simulink model "StateSpaceControl"  (R2023b)
settings: Solver=VariableStepAuto  StartTime=0.0  StopTime=20  RelTol=1e-3
values from neighbouring files (symbols this model uses):
  Time = 0:Delta:20    [Animation.m]    (also in Animation2.m; Animation3.m)
undefined symbols (not defined in the file or in its folder): A, B, C, Continuous, D, K_LQR
libraries: ctrlSharedLib x1
settings Model: Creator=BenWo  LastModifiedBy=BenWo

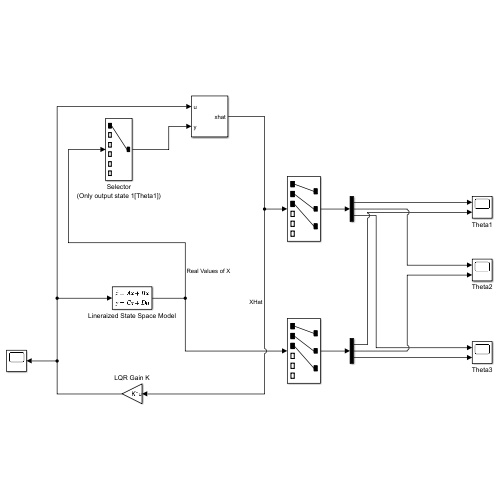
[thumbnail: Simulink's stored preview of the top-level diagram]
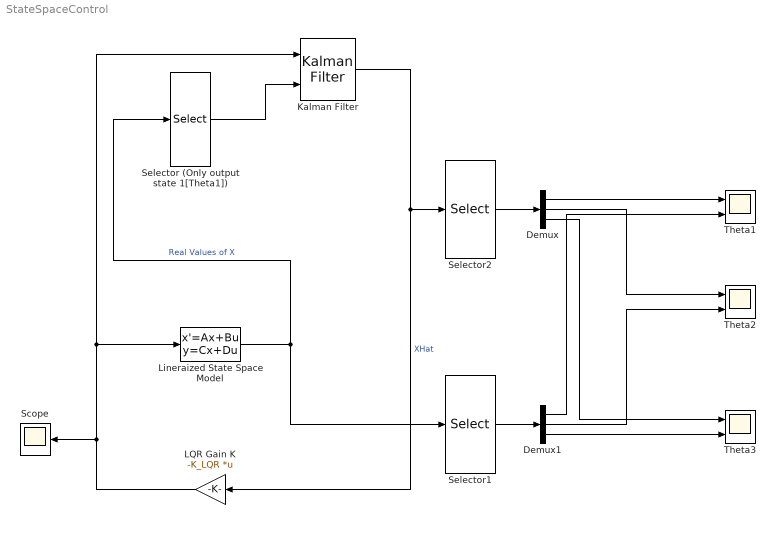
== system StateSpaceControl ==
  Demux : Demux  Outputs=3
  Demux1 : Demux  Outputs=3
  Kalman Filter : ctrlSharedLib/Kalman Filter  TimeDomain=Continuous-Time  UseCurrentEstimator=on  ModelSource=Individual A, B, C, D matrices  ModelSourceVariable=ss(0.95,1,1,0,1)  A=A  B=B  C=C  D=D  NumberOfStates=1  NumberOfInputs=1  NumberOfOutputs=1  InitialEstimateSource=Dialog  X0=0  P0=10  UseK=off  UseGH=off  NumberOfProcessNoiseInputs=1  G=1  TimeInvariantG=on  H=0  TimeInvariantH=on  Q=LQ  TimeInvariantQ=on  R=1  TimeInvariantR=on  N=0  TimeInvariantN=on  AddInputPort=on  AddEnablePort=off  OutputEstimatedY=off  OutputP=off  Ts=-1
  LQR Gain K : Gain  Gain=-K_LQR  Multiplication=Matrix(K*u)
  Lineraized State Space Model : StateSpace  A=A  B=B  C=eye(6)  D=zeros(6,1)  InitialCondition=[0,0.1,0,0,0,0]  ParameterTunability=Optimized
  Scope : Scope
  Selector (Only output state 1[Theta1]) : Selector  InputPortWidth=6  IndexOptions=Index vector (dialog)  Indices=[1]  OutputSizes=1
  Selector1 : Selector  InputPortWidth=6  IndexOptions=Index vector (dialog)  Indices=[1:3]  OutputSizes=1
  Selector2 : Selector  InputPortWidth=6  IndexOptions=Index vector (dialog)  Indices=[1:3]  OutputSizes=1
  Theta1 : Scope  NumInputPorts=2
  Theta2 : Scope  NumInputPorts=2
  Theta3 : Scope  NumInputPorts=2
  wires:
  Demux/1 -> Theta1/1
  Demux/2 -> Theta2/1
  Demux/3 -> Theta3/1
  Lineraized State Space Model/1 -> Selector1/1, Selector (Only output state 1[Theta1])/1  "Real Values of X"
  Selector1/1 -> Demux1/1
  Demux1/1 -> Theta1/2
  Demux1/2 -> Theta2/2
  Demux1/3 -> Theta3/2
  LQR Gain K/1 -> Scope/1, Lineraized State Space Model/1, Kalman Filter/1
  Kalman Filter/1 -> Selector2/1, LQR Gain K/1  "XHat"
  Selector2/1 -> Demux/1
  Selector (Only output state 1[Theta1])/1 -> Kalman Filter/2
